simulink model "TF_simulink"  (R2018b)
settings: Solver=VariableStepAuto  StartTime=0.0  StopTime=7  RelTol=1e-3
undefined symbols (not defined in the file): d, g, l, m
libraries: vrlib x4, simulink_extras x1
settings Model: Creator=ferra  LastModifiedBy=ferra

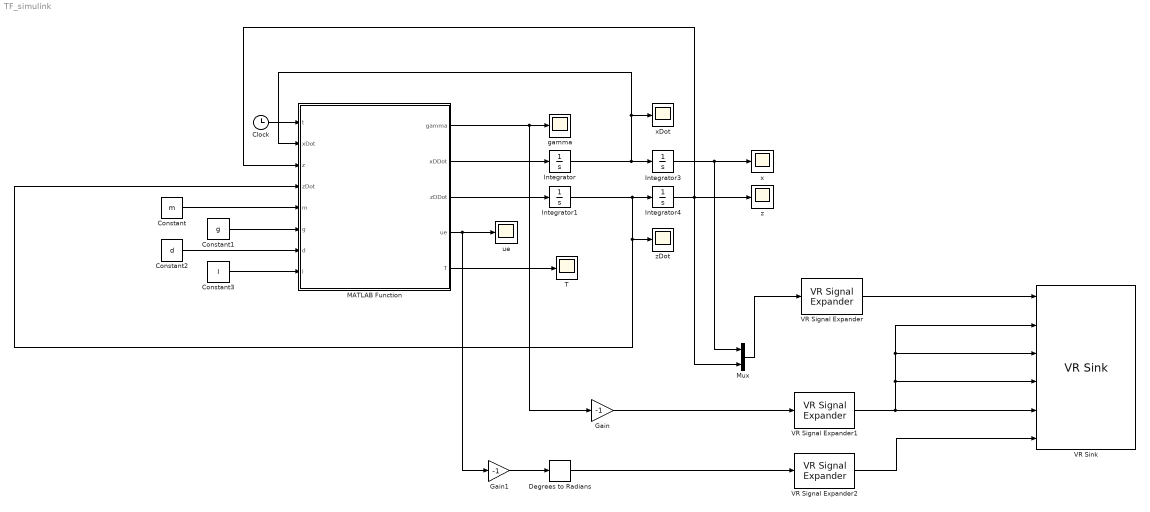
== system TF_simulink ==
  Clock : Clock
  Constant : Constant  Value=m
  Constant1 : Constant  Value=g
  Constant2 : Constant  Value=d
  Constant3 : Constant  Value=l
  Degrees to Radians : simulink_extras/Transformations/Degrees to Radians
  Gain : Gain  Gain=-1
  Gain1 : Gain  Gain=-1
  Integrator : Integrator
  Integrator1 : Integrator  InitialCondition=1
  Integrator3 : Integrator
  Integrator4 : Integrator
  MATLAB Function : MATLAB Function  TreatAsAtomicUnit=on
  Mux : Mux  Inputs=2
  T : Scope
  VR Signal Expander : vrlib/VR Signal Expander  outwidth=3  outidx=[1 2]
      settings: SourceProductName=Simulink 3D Animation  SourceProductBaseCode=VR
  VR Signal Expander1 : vrlib/VR Signal Expander  outwidth=4  outidx=[4]
      settings: SourceProductName=Simulink 3D Animation  SourceProductBaseCode=VR
  VR Signal Expander2 : vrlib/VR Signal Expander  outwidth=4  outidx=[4]
      settings: SourceProductName=Simulink 3D Animation  SourceProductBaseCode=VR
  VR Sink : vrlib/VR Sink  InstantiateOnLoad=on  SampleTime=0.01  ViewEnable=on  RemoteChange=off  RemoteView=off  FieldsWritten=Airplane.translation.3.1.1.double#Rotor_1.rotation.4.1.1.double#Rotor_2.rotation.4.1.1.double#Rotor_3.rotation.4.1.1.double#Rotor_4.rotation.4.1.1.double#Flap_tail.rotation.4.1.1.double  WorldFileName=C:\Users\ferra\Desktop\Projects\Matlab\Thesis\3D-simulation\3D_world.WRL  AutoView=off  VideoDimensions=[]  AllowVariableSize=off
      settings: SourceProductBaseCode=VR
  gamma : Scope
  ue : Scope
  x : Scope
  xDot : Scope
  z : Scope
  zDot : Scope
  wires:
  MATLAB Function/1(gamma) -> Gain/1, gamma/1
  Clock/1 -> MATLAB Function/1(t)
  MATLAB Function/2(xDDot) -> Integrator/1
  MATLAB Function/3(zDDot) -> Integrator1/1
  Integrator/1 -> MATLAB Function/2(xDot), xDot/1, Integrator3/1
  Integrator1/1 -> zDot/1, MATLAB Function/4(zDot), Integrator4/1
  Constant/1 -> MATLAB Function/5(m)
  Constant1/1 -> MATLAB Function/6(g)
  Constant2/1 -> MATLAB Function/7(d)
  Constant3/1 -> MATLAB Function/8(l)
  Integrator3/1 -> x/1, Mux/1
  Integrator4/1 -> Mux/2, z/1, MATLAB Function/3(z)
  MATLAB Function/5(T) -> T/1
  Mux/1 -> VR Signal Expander/1
  Gain/1 -> VR Signal Expander1/1
  Degrees to Radians/1 -> VR Signal Expander2/1
  Gain1/1 -> Degrees to Radians/1
  MATLAB Function/4(ue) -> Gain1/1, ue/1
  VR Signal Expander1/1 -> VR Sink/4, VR Sink/2, VR Sink/3, VR Sink/5
  VR Signal Expander2/1 -> VR Sink/6
  VR Signal Expander/1 -> VR Sink/1

== matlab function TF_simulink/MATLAB Function ==
  data: t input; gamma output; xDDot output; zDDot output; ue output; xDot input; z input; zDot input; m input; g input; d input; l input; T output
function [gamma,xDDot,zDDot,ue, T] = TF(t,xDot,z,zDot,m,g,d,l)

ue = 0;
zDes = 10;
kpz = 10;
kdz = 4;

k1 = 2;
k2 = 3;


T = 10;


drag = -d * xDot^2;
lift = l * xDot^2;


%virtual controller
vz = kpz*(z-zDes)+kdz*zDot;

phi = -k1*(z-zDes);
e1 = zDot-phi;
phiDot = -k1*(e1  + k1*(z-zDes));


%Change angle of thrusts
gamma =t/2;
if(abs(gamma)> pi/2)
   gamma = pi/2; 
end


%Check if lift force > mg
if(lift-m*g>0 && abs(gamma)>deg2rad(85) )
    ue = -(T*cos(gamma)+l*xDot^2-m*g+vz)/(xDot^2);

elseif(abs(gamma)< deg2rad(85))
    T = (-z - lift +m*g+phiDot-k2*e1)/(cos(gamma));
end


xDDot = T*sin(gamma) + drag;
zDDot = T*cos(gamma) + lift + ue*xDot^2 -m*g;



end
